simulink model "CPS_PowerSync_System"  (R2024a)
settings: Solver=FixedStepAuto  StartTime=0.0  StopTime=50  FixedStep=0.1  RelTol=1e-3
model workspace (MAT data in the model file):
  SoC : Simulink.Signal (value not decoded)
undefined symbols (not defined in the file or in its folder): m, v_CP1, v_CP2, v_CP3, w_CP1, w_CP2, w_CP3
(part 2 of 3)

== system CPS_PowerSync_System/ElecritcVehicles3/Normal.Plugged.Completed ==
  Action Port : ActionPort
      settings: CopyFcn=Stateflow.SLINSF.SimulinkMan.removeBlockPreDeleteFcn  PreDeleteFcn=Stateflow.SLINSF.SimulinkMan.unsafePredeleteFcn
  Constant : Constant
  If Action Subsystem : Subsystem  TreatAsAtomicUnit=on
  Switch Case : SwitchCase
  plug : Outport
  powerRequest : Outport  Port=2
  wires:
  Constant/1 -> Switch Case/1
  Switch Case/1 -> If Action Subsystem/Action
  If Action Subsystem/1(plug) -> plug/1
  If Action Subsystem/2(powerRequest) -> powerRequest/1

== system CPS_PowerSync_System/ElecritcVehicles3/Normal.Unplugged.Assigment ==
  powerFlow : Inport
  Action Port : ActionPort
      settings: CopyFcn=Stateflow.SLINSF.SimulinkMan.removeBlockPreDeleteFcn  PreDeleteFcn=Stateflow.SLINSF.SimulinkMan.unsafePredeleteFcn
  Constant : Constant  Value=0  OutDataTypeStr=boolean
  powerRequest : Outport
  plug : Outport  Port=2
  wires:
  Constant/1 -> powerRequest/1, plug/1

== system CPS_PowerSync_System/Simulink Function ==
  get_event_CP1 : TriggerPort  TriggerType=function-call  IsSimulinkFunction=on  FunctionName=get_event_CP1  FunctionVisibility=scoped  VariantControl=(inherit)
  Constant : Constant
  Send : Send  OutputPortMessageModes=m
  Out1 : Outport
  wires:
  Constant/1 -> Send/1
  Send/1 -> Out1/1

== system CPS_PowerSync_System/Simulink Function1 ==
  get_event_CP2 : TriggerPort  TriggerType=function-call  IsSimulinkFunction=on  FunctionName=get_event_CP2  FunctionVisibility=scoped  VariantControl=(inherit)
  Constant : Constant
  Send : Send  OutputPortMessageModes=m
  Out1 : Outport
  wires:
  Send/1 -> Out1/1
  Constant/1 -> Send/1

== system CPS_PowerSync_System/Simulink Function2 ==
  dead_CP2 : TriggerPort  TriggerType=function-call  IsSimulinkFunction=on  FunctionName=dead_CP2  FunctionVisibility=scoped  VariantControl=(inherit)
  Constant : Constant  Value=2
  Send : Send  OutputPortMessageModes=m
  Out1 : Outport
  wires:
  Constant/1 -> Send/1
  Send/1 -> Out1/1

== system CPS_PowerSync_System/Simulink Function3 ==
  response_2_to_1 : TriggerPort  TriggerType=function-call  IsSimulinkFunction=on  FunctionName=response_2_to_1  FunctionVisibility=scoped  VariantControl=(inherit)
  Constant : Constant  Value=3
  Send : Send  OutputPortMessageModes=m
  Out1 : Outport
  wires:
  Constant/1 -> Send/1
  Send/1 -> Out1/1

== system CPS_PowerSync_System/Simulink Function4 ==
  response_3_to_2 : TriggerPort  TriggerType=function-call  IsSimulinkFunction=on  FunctionName=response_3_to_2  FunctionVisibility=scoped  VariantControl=(inherit)
  Constant : Constant  Value=3
  Send : Send  OutputPortMessageModes=m
  Out1 : Outport
  wires:
  Send/1 -> Out1/1
  Constant/1 -> Send/1

== system CPS_PowerSync_System/Simulink Function5 ==
  elected_CP3 : TriggerPort  TriggerType=function-call  IsSimulinkFunction=on  FunctionName=elected_CP3  FunctionVisibility=scoped  VariantControl=(inherit)
  Constant : Constant  Value=3
  Send : Send  OutputPortMessageModes=m
  Out1 : Outport
  wires:
  Constant/1 -> Send/1
  Send/1 -> Out1/1

== system CPS_PowerSync_System/Simulink Function6 ==
  elected_CP2 : TriggerPort  TriggerType=function-call  IsSimulinkFunction=on  FunctionName=elected_CP2  FunctionVisibility=scoped  VariantControl=(inherit)
  Constant : Constant  Value=2
  Send : Send  OutputPortMessageModes=m
  Out1 : Outport
  wires:
  Constant/1 -> Send/1
  Send/1 -> Out1/1

== system CPS_PowerSync_System/Simulink Function7 ==
  dead_CP1 : TriggerPort  TriggerType=function-call  IsSimulinkFunction=on  FunctionName=dead_CP1  FunctionVisibility=scoped  VariantControl=(inherit)
  Constant : Constant  Value=2
  Send : Send  OutputPortMessageModes=m
  Out1 : Outport
  wires:
  Constant/1 -> Send/1
  Send/1 -> Out1/1

== system CPS_PowerSync_System/Simulink Function8 ==
  dead_CP3 : TriggerPort  TriggerType=function-call  IsSimulinkFunction=on  FunctionName=dead_CP3  FunctionVisibility=scoped  VariantControl=(inherit)
  Constant : Constant  Value=2
  Send : Send  OutputPortMessageModes=m
  Out1 : Outport
  wires:
  Constant/1 -> Send/1
  Send/1 -> Out1/1

== system CPS_PowerSync_System/Simulink Function9 ==
  response_3_to_1 : TriggerPort  TriggerType=function-call  IsSimulinkFunction=on  FunctionName=response_3_to_1  FunctionVisibility=scoped  VariantControl=(inherit)
  Constant : Constant  Value=3
  Send : Send  OutputPortMessageModes=m
  Out1 : Outport
  wires:
  Constant/1 -> Send/1
  Send/1 -> Out1/1

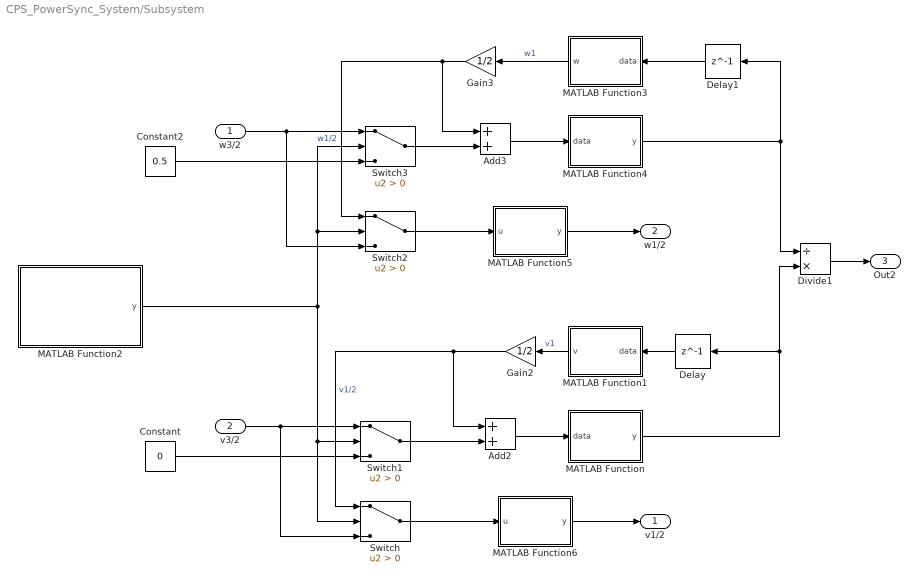
== system CPS_PowerSync_System/Subsystem ==
  w3/2 : Inport  SampleTime=0.1
  v3/2 : Inport  Port=2  SampleTime=0.1
  Add2 : Sum
  Add3 : Sum
  Constant : Constant  Value=0  SampleTime=0.1
  Constant2 : Constant  Value=0.5  SampleTime=0.1
  Delay : Delay  DelayLength=1  InitialCondition=v_CP1  SampleTime=0.1
  Delay1 : Delay  DelayLength=1  InitialCondition=w_CP1  SampleTime=0.1
  Divide1 : Product  Inputs=/*
  Gain2 : Gain  Gain=1/2
  Gain3 : Gain  Gain=1/2
  MATLAB Function : MATLAB Function  TreatAsAtomicUnit=on
  MATLAB Function1 : MATLAB Function  TreatAsAtomicUnit=on
  MATLAB Function2 : MATLAB Function  TreatAsAtomicUnit=on
  MATLAB Function3 : MATLAB Function  TreatAsAtomicUnit=on
  MATLAB Function4 : MATLAB Function  TreatAsAtomicUnit=on
  MATLAB Function5 : MATLAB Function  TreatAsAtomicUnit=on
  MATLAB Function6 : MATLAB Function  TreatAsAtomicUnit=on
  Switch{,1..3} (4 alike) : Switch  Criteria=u2 > Threshold  SaturateOnIntegerOverflow=off  InputSameDT=off
  v1/2 : Outport  SampleTime=0.1
  w1/2 : Outport  Port=2  SampleTime=0.1  VectorParamsAs1DForOutWhenUnconnected=off
  Out2 : Outport  Port=3  OutDataTypeStr=double  SampleTime=0.1
  wires:
  Gain3/1 -> Add3/1, Switch2/1  "w1/2"
  MATLAB Function1/1(v) -> Gain2/1  "v1"
  MATLAB Function2/1(y) -> Switch3/2, Switch2/2, Switch/2, Switch1/2
  Constant/1 -> Switch1/3
  Add3/1 -> MATLAB Function4/1(data)
  v3/2/1 -> Switch1/1, Switch/3
  Switch3/1 -> Add3/2
  MATLAB Function3/1(w) -> Gain3/1  "w1"
  Gain2/1 -> Switch/1, Add2/1  "v1/2"
  Switch1/1 -> Add2/2
  w3/2/1 -> Switch3/1, Switch2/3
  Delay/1 -> MATLAB Function1/1(data)
  Add2/1 -> MATLAB Function/1(data)
  MATLAB Function/1(y) -> Delay/1, Divide1/2
  Divide1/1 -> Out2/1
  Delay1/1 -> MATLAB Function3/1(data)
  MATLAB Function4/1(y) -> Delay1/1, Divide1/1
  Constant2/1 -> Switch3/3
  MATLAB Function5/1(y) -> w1/2/1
  MATLAB Function6/1(y) -> v1/2/1
  Switch2/1 -> MATLAB Function5/1(u)
  Switch/1 -> MATLAB Function6/1(u)

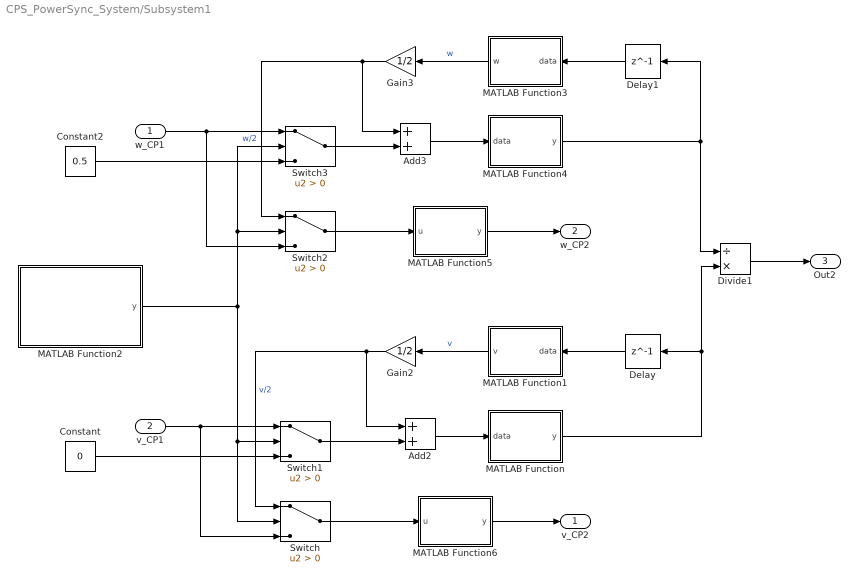
== system CPS_PowerSync_System/Subsystem1 ==
  w_CP1 : Inport  SampleTime=0.1
  v_CP1 : Inport  Port=2  SampleTime=0.1
  Add2 : Sum
  Add3 : Sum
  Constant : Constant  Value=0  SampleTime=0.1
  Constant2 : Constant  Value=0.5  SampleTime=0.1
  Delay : Delay  DelayLength=1  InitialCondition=v_CP2  SampleTime=0.1
  Delay1 : Delay  DelayLength=1  InitialCondition=w_CP2  SampleTime=0.1
  Divide1 : Product  Inputs=/*
  Gain2 : Gain  Gain=1/2
  Gain3 : Gain  Gain=1/2
  MATLAB Function : MATLAB Function  TreatAsAtomicUnit=on
  MATLAB Function1 : MATLAB Function  TreatAsAtomicUnit=on
  MATLAB Function2 : MATLAB Function  TreatAsAtomicUnit=on
  MATLAB Function3 : MATLAB Function  TreatAsAtomicUnit=on
  MATLAB Function4 : MATLAB Function  TreatAsAtomicUnit=on
  MATLAB Function5 : MATLAB Function  TreatAsAtomicUnit=on
  MATLAB Function6 : MATLAB Function  TreatAsAtomicUnit=on
  Switch{,1..3} (4 alike) : Switch  Criteria=u2 > Threshold  SaturateOnIntegerOverflow=off  InputSameDT=off
  v_CP2 : Outport  SampleTime=0.1
  w_CP2 : Outport  Port=2  SampleTime=0.1  VectorParamsAs1DForOutWhenUnconnected=off
  Out2 : Outport  Port=3  OutDataTypeStr=double  SampleTime=0.1
  wires:
  Gain3/1 -> Add3/1, Switch2/1  "w/2"
  MATLAB Function1/1(v) -> Gain2/1  "v"
  MATLAB Function2/1(y) -> Switch3/2, Switch2/2, Switch/2, Switch1/2
  Constant/1 -> Switch1/3
  Add3/1 -> MATLAB Function4/1(data)
  v_CP1/1 -> Switch1/1, Switch/3
  Switch3/1 -> Add3/2
  MATLAB Function3/1(w) -> Gain3/1  "w"
  Gain2/1 -> Switch/1, Add2/1  "v/2"
  Switch1/1 -> Add2/2
  w_CP1/1 -> Switch3/1, Switch2/3
  Delay/1 -> MATLAB Function1/1(data)
  Add2/1 -> MATLAB Function/1(data)
  MATLAB Function/1(y) -> Delay/1, Divide1/2
  Divide1/1 -> Out2/1
  Delay1/1 -> MATLAB Function3/1(data)
  MATLAB Function4/1(y) -> Delay1/1, Divide1/1
  Constant2/1 -> Switch3/3
  MATLAB Function5/1(y) -> w_CP2/1
  MATLAB Function6/1(y) -> v_CP2/1
  Switch2/1 -> MATLAB Function5/1(u)
  Switch/1 -> MATLAB Function6/1(u)

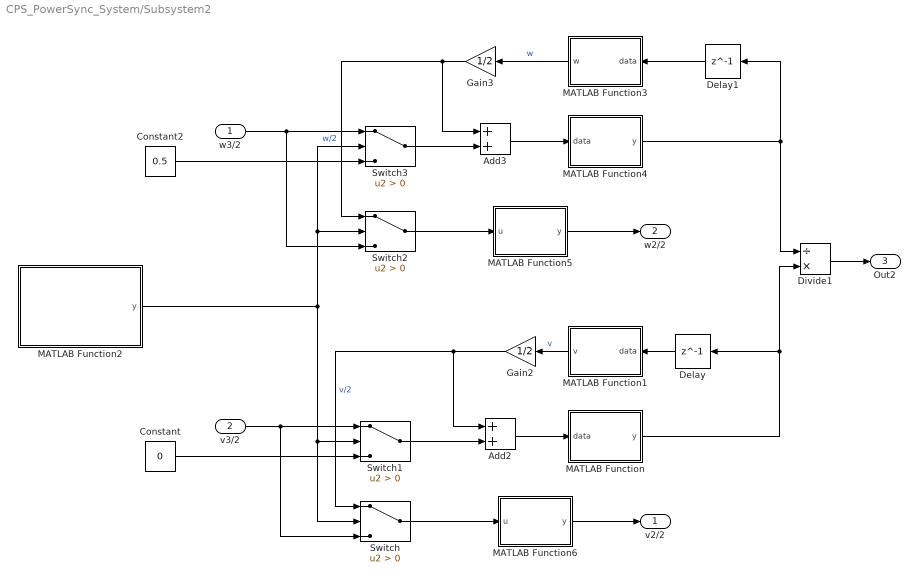
== system CPS_PowerSync_System/Subsystem2 ==
  w3/2 : Inport  SampleTime=0.1
  v3/2 : Inport  Port=2  SampleTime=0.1
  Add2 : Sum
  Add3 : Sum
  Constant : Constant  Value=0  SampleTime=0.1
  Constant2 : Constant  Value=0.5  SampleTime=0.1
  Delay : Delay  DelayLength=1  InitialCondition=v_CP3  SampleTime=0.1
  Delay1 : Delay  DelayLength=1  InitialCondition=w_CP3  SampleTime=0.1
  Divide1 : Product  Inputs=/*
  Gain2 : Gain  Gain=1/2
  Gain3 : Gain  Gain=1/2
  MATLAB Function : MATLAB Function  TreatAsAtomicUnit=on
  MATLAB Function1 : MATLAB Function  TreatAsAtomicUnit=on
  MATLAB Function2 : MATLAB Function  TreatAsAtomicUnit=on
  MATLAB Function3 : MATLAB Function  TreatAsAtomicUnit=on
  MATLAB Function4 : MATLAB Function  TreatAsAtomicUnit=on
  MATLAB Function5 : MATLAB Function  TreatAsAtomicUnit=on
  MATLAB Function6 : MATLAB Function  TreatAsAtomicUnit=on
  Switch{,1..3} (4 alike) : Switch  Criteria=u2 > Threshold  SaturateOnIntegerOverflow=off  InputSameDT=off
  v2/2 : Outport  SampleTime=0.1
  w2/2 : Outport  Port=2  SampleTime=0.1  VectorParamsAs1DForOutWhenUnconnected=off
  Out2 : Outport  Port=3  OutDataTypeStr=double  SampleTime=0.1
  wires:
  Gain3/1 -> Add3/1, Switch2/1  "w/2"
  MATLAB Function1/1(v) -> Gain2/1  "v"
  MATLAB Function2/1(y) -> Switch3/2, Switch2/2, Switch/2, Switch1/2
  Constant/1 -> Switch1/3
  Add3/1 -> MATLAB Function4/1(data)
  v3/2/1 -> Switch1/1, Switch/3
  Switch3/1 -> Add3/2
  MATLAB Function3/1(w) -> Gain3/1  "w"
  Gain2/1 -> Switch/1, Add2/1  "v/2"
  Switch1/1 -> Add2/2
  w3/2/1 -> Switch3/1, Switch2/3
  Delay/1 -> MATLAB Function1/1(data)
  Add2/1 -> MATLAB Function/1(data)
  MATLAB Function/1(y) -> Delay/1, Divide1/2
  Divide1/1 -> Out2/1
  Delay1/1 -> MATLAB Function3/1(data)
  MATLAB Function4/1(y) -> Delay1/1, Divide1/1
  Constant2/1 -> Switch3/3
  MATLAB Function5/1(y) -> w2/2/1
  MATLAB Function6/1(y) -> v2/2/1
  Switch2/1 -> MATLAB Function5/1(u)
  Switch/1 -> MATLAB Function6/1(u)

== system CPS_PowerSync_System/WirelessReceiveModule ==
  Bus Selector : BusSelector  OutputSignals=v3/2,w3/2
  Multicast Receive Queue : Queue  OutputPortMessageModes=m  EntityArrivalSource=Multicast  MulticastTag=F
  Receive : Receive  InputPortMessageModes=m  UseInternalQueue=off  QueueOverwriting=on  QueueLength=1  QueueType=LIFO  SampleTime=0.1
  <w3/2> : Outport  SampleTime=0.1
  <v3/2> : Outport  Port=2  SampleTime=0.1
  wires:
  Receive/1 -> Bus Selector/1
  Bus Selector/1 -> <v3/2>/1  "<v3/2>"
  Bus Selector/2 -> <w3/2>/1  "<w3/2>"
  Multicast Receive Queue/1 -> Receive/1

== system CPS_PowerSync_System/WirelessReceiveModule1 ==
  Bus Selector : BusSelector  OutputSignals=w1/2,v1/2
  Multicast Receive Queue : Queue  OutputPortMessageModes=m  EntityArrivalSource=Multicast  MulticastTag=D
  Receive : Receive  InputPortMessageModes=m  UseInternalQueue=off  QueueOverwriting=on  QueueLength=1  QueueType=LIFO
  <w1/2> : Outport  SampleTime=0.1
  <v1/2> : Outport  Port=2  SampleTime=0.1
  wires:
  Bus Selector/2 -> <v1/2>/1  "<v1/2>"
  Multicast Receive Queue/1 -> Receive/1
  Receive/1 -> Bus Selector/1
  Bus Selector/1 -> <w1/2>/1  "<w1/2>"

== system CPS_PowerSync_System/WirelessReceiveModule2 ==
  Bus Selector : BusSelector  OutputSignals=v2/2,w2/2
  Multicast Receive Queue : Queue  OutputPortMessageModes=m  EntityArrivalSource=Multicast  MulticastTag=E
  Receive : Receive  InputPortMessageModes=m  UseInternalQueue=off  QueueOverwriting=on  QueueLength=1  QueueType=LIFO
  <w2/2> : Outport  SampleTime=0.1
  <v2/2> : Outport  Port=2  SampleTime=0.1
  wires:
  Bus Selector/2 -> <w2/2>/1  "<w2/2>"
  Multicast Receive Queue/1 -> Receive/1
  Receive/1 -> Bus Selector/1
  Bus Selector/1 -> <v2/2>/1  "<v2/2>"

== system CPS_PowerSync_System/WirelessSendModule ==
  v1/2 : Inport  SampleTime=0.1
  w1/2 : Inport  Port=2  SampleTime=0.1
  Bus Creator : BusCreator  Inputs=2  OutDataTypeStr=Bus: BusObject  NonVirtualBus=on
  Entity Multicast : EntityMulticast  Tag=D  InputPortMessageModes=m  MulticastTag=D
  Send : Send  OutputPortMessageModes=m
  wires:
  Send/1 -> Entity Multicast/1
  Bus Creator/1 -> Send/1
  v1/2/1 -> Bus Creator/2  "v1/2"
  w1/2/1 -> Bus Creator/1  "w1/2"

== system CPS_PowerSync_System/WirelessSendModule1 ==
  v2/2 : Inport  SampleTime=0.1
  w2/2 : Inport  Port=2  SampleTime=0.1
  Bus Creator : BusCreator  Inputs=2  OutDataTypeStr=Bus: BusObject  NonVirtualBus=on
  Entity Multicast : EntityMulticast  Tag=E  InputPortMessageModes=m  MulticastTag=E
  Send : Send  OutputPortMessageModes=m
  wires:
  Bus Creator/1 -> Send/1
  Send/1 -> Entity Multicast/1
  v2/2/1 -> Bus Creator/1  "v2/2"
  w2/2/1 -> Bus Creator/2  "w2/2"

== system CPS_PowerSync_System/WirelessSendModule2 ==
  v3/2 : Inport  SampleTime=0.1
  w3/2 : Inport  Port=2  SampleTime=0.1
  Bus Creator : BusCreator  Inputs=2  OutDataTypeStr=Bus: BusObject  NonVirtualBus=on
  Entity Multicast : EntityMulticast  Tag=F  InputPortMessageModes=m  MulticastTag=F
  Send : Send  OutputPortMessageModes=m
  wires:
  Bus Creator/1 -> Send/1
  v3/2/1 -> Bus Creator/1  "v3/2"
  w3/2/1 -> Bus Creator/2  "w3/2"
  Send/1 -> Entity Multicast/1

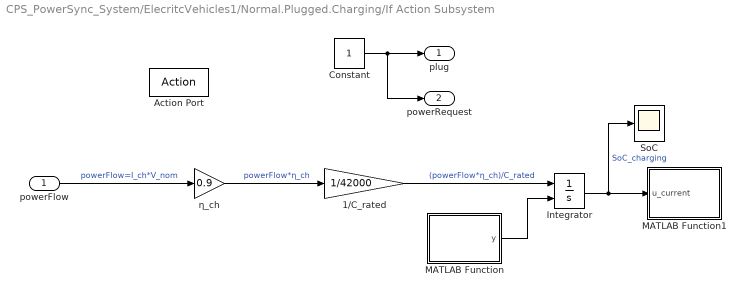
== system CPS_PowerSync_System/ElecritcVehicles1/Normal.Plugged.Charging/If Action Subsystem ==
  powerFlow : Inport
  Action Port : ActionPort  InitializeStates=reset  ActionPortLabel=case [ 1 ]:
  1/C_rated : Gain  Gain=1/42000
  Constant : Constant  OutDataTypeStr=boolean
  Integrator : Integrator  InitialConditionSource=external  LimitOutput=on  UpperSaturationLimit=1  LowerSaturationLimit=0
  MATLAB Function : MATLAB Function  TreatAsAtomicUnit=on
  MATLAB Function1 : MATLAB Function  TreatAsAtomicUnit=on
  SoC : Scope
  η_ch : Gain  Gain=0.9
  plug : Outport  OutDataTypeStr=boolean
  powerRequest : Outport  Port=2  OutDataTypeStr=boolean
  wires:
  1/C_rated/1 -> Integrator/1  "(powerFlow*η_ch)/C_rated"
  η_ch/1 -> 1/C_rated/1  "powerFlow*η_ch"
  Constant/1 -> plug/1, powerRequest/1
  Integrator/1 -> SoC/1, MATLAB Function1/1(u_current)  "SoC_charging"
  powerFlow/1 -> η_ch/1  "powerFlow=I_ch*V_nom"
  MATLAB Function/1(y) -> Integrator/2

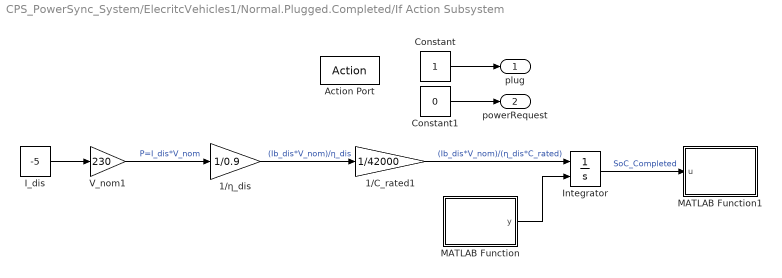
== system CPS_PowerSync_System/ElecritcVehicles1/Normal.Plugged.Completed/If Action Subsystem ==
  Action Port : ActionPort  InitializeStates=reset  ActionPortLabel=case [ 1 ]:
  1/C_rated1 : Gain  Gain=1/42000
  1/η_dis : Gain  Gain=1/0.9
  Constant : Constant  OutDataTypeStr=boolean
  Constant1 : Constant  Value=0  OutDataTypeStr=boolean
  I_dis : Constant  Value=-5
  Integrator : Integrator  InitialConditionSource=external  LimitOutput=on  UpperSaturationLimit=1  LowerSaturationLimit=0
  MATLAB Function : MATLAB Function  TreatAsAtomicUnit=on
  MATLAB Function1 : MATLAB Function  TreatAsAtomicUnit=on
  V_nom1 : Gain  Gain=230
  plug : Outport  OutDataTypeStr=boolean
  powerRequest : Outport  Port=2  OutDataTypeStr=boolean
  wires:
  Integrator/1 -> MATLAB Function1/1(u)  "SoC_Completed"
  MATLAB Function/1(y) -> Integrator/2
  Constant1/1 -> powerRequest/1
  1/η_dis/1 -> 1/C_rated1/1  "(Ib_dis*V_nom)/η_dis"
  V_nom1/1 -> 1/η_dis/1  "P=I_dis*V_nom"
  1/C_rated1/1 -> Integrator/1  "(Ib_dis*V_nom)/(η_dis*C_rated)"
  I_dis/1 -> V_nom1/1
  Constant/1 -> plug/1

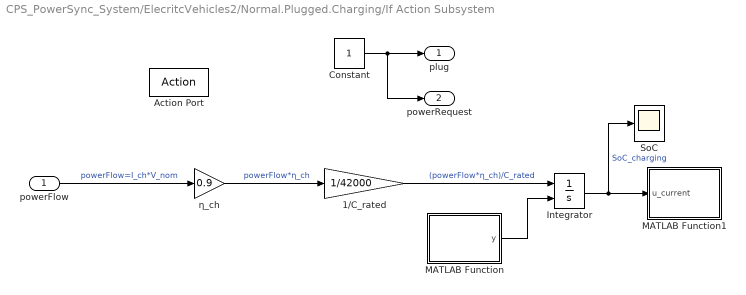
== system CPS_PowerSync_System/ElecritcVehicles2/Normal.Plugged.Charging/If Action Subsystem ==
  powerFlow : Inport
  Action Port : ActionPort  InitializeStates=reset  ActionPortLabel=case [ 1 ]:
  1/C_rated : Gain  Gain=1/42000
  Constant : Constant  OutDataTypeStr=boolean
  Integrator : Integrator  InitialConditionSource=external  LimitOutput=on  UpperSaturationLimit=1  LowerSaturationLimit=0
  MATLAB Function : MATLAB Function  TreatAsAtomicUnit=on
  MATLAB Function1 : MATLAB Function  TreatAsAtomicUnit=on
  SoC : Scope
  η_ch : Gain  Gain=0.9
  plug : Outport  OutDataTypeStr=boolean
  powerRequest : Outport  Port=2  OutDataTypeStr=boolean
  wires:
  MATLAB Function/1(y) -> Integrator/2
  powerFlow/1 -> η_ch/1  "powerFlow=I_ch*V_nom"
  Integrator/1 -> MATLAB Function1/1(u_current), SoC/1  "SoC_charging"
  Constant/1 -> powerRequest/1, plug/1
  η_ch/1 -> 1/C_rated/1  "powerFlow*η_ch"
  1/C_rated/1 -> Integrator/1  "(powerFlow*η_ch)/C_rated"

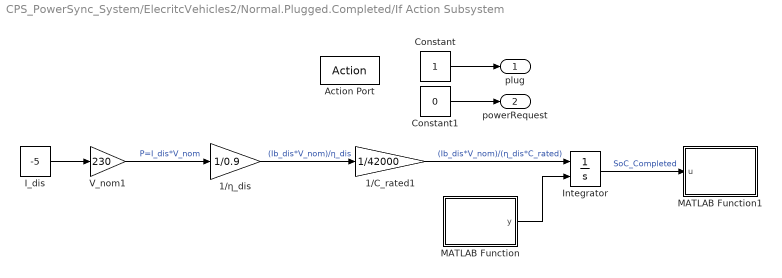
== system CPS_PowerSync_System/ElecritcVehicles2/Normal.Plugged.Completed/If Action Subsystem ==
  Action Port : ActionPort  InitializeStates=reset  ActionPortLabel=case [ 1 ]:
  1/C_rated1 : Gain  Gain=1/42000
  1/η_dis : Gain  Gain=1/0.9
  Constant : Constant  OutDataTypeStr=boolean
  Constant1 : Constant  Value=0  OutDataTypeStr=boolean
  I_dis : Constant  Value=-5
  Integrator : Integrator  InitialConditionSource=external  LimitOutput=on  UpperSaturationLimit=1  LowerSaturationLimit=0
  MATLAB Function : MATLAB Function  TreatAsAtomicUnit=on
  MATLAB Function1 : MATLAB Function  TreatAsAtomicUnit=on
  V_nom1 : Gain  Gain=230
  plug : Outport  OutDataTypeStr=boolean
  powerRequest : Outport  Port=2  OutDataTypeStr=boolean
  wires:
  Constant/1 -> plug/1
  I_dis/1 -> V_nom1/1
  1/C_rated1/1 -> Integrator/1  "(Ib_dis*V_nom)/(η_dis*C_rated)"
  V_nom1/1 -> 1/η_dis/1  "P=I_dis*V_nom"
  1/η_dis/1 -> 1/C_rated1/1  "(Ib_dis*V_nom)/η_dis"
  Constant1/1 -> powerRequest/1
  MATLAB Function/1(y) -> Integrator/2
  Integrator/1 -> MATLAB Function1/1(u)  "SoC_Completed"

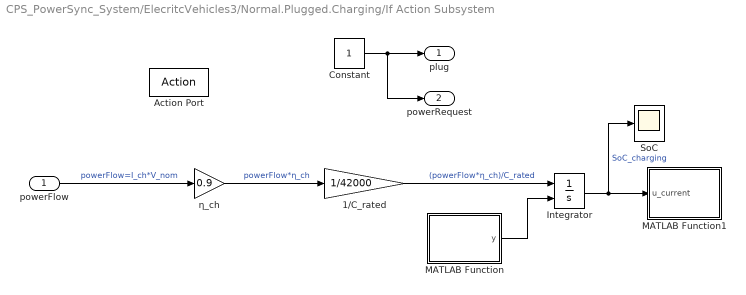
== system CPS_PowerSync_System/ElecritcVehicles3/Normal.Plugged.Charging/If Action Subsystem ==
  powerFlow : Inport
  Action Port : ActionPort  InitializeStates=reset  ActionPortLabel=case [ 1 ]:
  1/C_rated : Gain  Gain=1/42000
  Constant : Constant  OutDataTypeStr=boolean
  Integrator : Integrator  InitialConditionSource=external  LimitOutput=on  UpperSaturationLimit=1  LowerSaturationLimit=0
  MATLAB Function : MATLAB Function  TreatAsAtomicUnit=on
  MATLAB Function1 : MATLAB Function  TreatAsAtomicUnit=on
  SoC : Scope
  η_ch : Gain  Gain=0.9
  plug : Outport  OutDataTypeStr=boolean
  powerRequest : Outport  Port=2  OutDataTypeStr=boolean
  wires:
  1/C_rated/1 -> Integrator/1  "(powerFlow*η_ch)/C_rated"
  η_ch/1 -> 1/C_rated/1  "powerFlow*η_ch"
  Constant/1 -> plug/1, powerRequest/1
  Integrator/1 -> SoC/1, MATLAB Function1/1(u_current)  "SoC_charging"
  powerFlow/1 -> η_ch/1  "powerFlow=I_ch*V_nom"
  MATLAB Function/1(y) -> Integrator/2

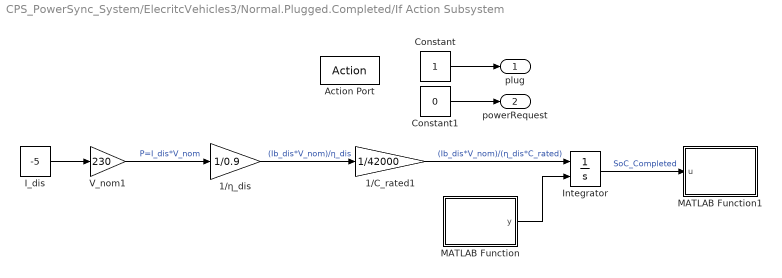
== system CPS_PowerSync_System/ElecritcVehicles3/Normal.Plugged.Completed/If Action Subsystem ==
  Action Port : ActionPort  InitializeStates=reset  ActionPortLabel=case [ 1 ]:
  1/C_rated1 : Gain  Gain=1/42000
  1/η_dis : Gain  Gain=1/0.9
  Constant : Constant  OutDataTypeStr=boolean
  Constant1 : Constant  Value=0  OutDataTypeStr=boolean
  I_dis : Constant  Value=-5
  Integrator : Integrator  InitialConditionSource=external  LimitOutput=on  UpperSaturationLimit=1  LowerSaturationLimit=0
  MATLAB Function : MATLAB Function  TreatAsAtomicUnit=on
  MATLAB Function1 : MATLAB Function  TreatAsAtomicUnit=on
  V_nom1 : Gain  Gain=230
  plug : Outport  OutDataTypeStr=boolean
  powerRequest : Outport  Port=2  OutDataTypeStr=boolean
  wires:
  Integrator/1 -> MATLAB Function1/1(u)  "SoC_Completed"
  MATLAB Function/1(y) -> Integrator/2
  Constant1/1 -> powerRequest/1
  1/η_dis/1 -> 1/C_rated1/1  "(Ib_dis*V_nom)/η_dis"
  V_nom1/1 -> 1/η_dis/1  "P=I_dis*V_nom"
  1/C_rated1/1 -> Integrator/1  "(Ib_dis*V_nom)/(η_dis*C_rated)"
  I_dis/1 -> V_nom1/1
  Constant/1 -> plug/1

== matlab function CPS_PowerSync_System/CP1 ==
  settings: updateMethod=DISCRETE  sampleTime=0.1
  data: clock input
function fcn(clock)

    % Funzioni per interagire con base workspace
    coder.extrinsic('evalin');
    coder.extrinsic('assignin');
    
    check_variables('flg_response_CP1');
    check_variables('t_send_CP1');
    check_variables('flg_send_CP1');
    check_variables('pr_previous_CP1');
    check_variables('pr_actual_CP1');
    
    % Aggiornamento del clock del CP1
    assignin('base', 'clock_CP1', clock);
    
    % Lettura variabili dal WS
    pr_previous = boolean(0); pr_actual = boolean(0); t_send = 0;
    pr_previous = evalin('base', 'boolean(pr_previous_CP1)');
    pr_actual = evalin('base', 'boolean(pr_actual_CP1)');
    t_send = evalin('base', 'double(t_send_CP1)');
    flg_response = evalin('base', 'boolean(flg_response_CP1)');
    flg_send = evalin('base', 'boolean(flg_send_CP1)');


    % Controllo se un veicolo si è connesso / disconnesso
    if pr_previous ~= pr_actual

        if pr_actual
            disp('CP1 requires power, so the leader must be re-elected.')
        else
            disp('CP1 requires no additional power, so the leader must be re-elected.')
        end
        
        dead_CP1();

    end

    % Controllo se mi è possibile diventare leader:

    % Tempo trascorso dall'invio del messaggio da parte del nodo 1
    t_elapsed = clock - t_send; 

    % Definizione del tempo da attendere per elezione leader
    delta = 1;
    
    % Se dopo delta secondi dal momento in cui ho inviato il messaggio
    % (t_elapsed >= delta) non ho ancora ricevuto una risposta
    % (~flg_response) e il mio flag_inviato non è stato resettato a zero
    % e ho il veicolo connesso, allora sarò il leader
    if t_elapsed >= delta && ~flg_response && flg_send && pr_actual

        % Il nodo 1 diventa leader
        assignin('base', 'v_CP1', 1);

        % Il nodo sa che il leader è stato eletto
        assignin('base', 'flg_elected_CP1', 1);

        disp('CP1 did not receive an answer, so it can declare itself leader.')

        % Elezione avvenuta
        % Tutti e tre questi flag sono necessari al corretto funzionamento dell'algoritmo push-sum
        assignin('base', 'flg_elected_CP1', 1);
        assignin('base', 'flg_first_instant_v_CP1', 1);
        assignin('base', 'flg_first_instant_w_CP1', 1);
    
        assignin('base', 'flg_send_CP1', 0);
        
        disp('CP1 is active and knows that the leader has been elected.')
        
    end

end

== matlab function CPS_PowerSync_System/CP2 ==
  settings: updateMethod=DISCRETE  sampleTime=0.1
  data: clock input
function fcn(clock)

    % Funzioni per interagire con base workspace
    coder.extrinsic('evalin');
    coder.extrinsic('assignin');
    
    check_variables('flg_response_CP2');
    check_variables('t_send_CP2');
    check_variables('flg_send_CP2');
    check_variables('pr_previous_CP2');
    check_variables('pr_actual_CP2');
    
    % Aggiornamento del clock del CP2
    assignin('base', 'clock_CP2', clock);
    
    % Lettura variabili dal WS
    pr_previous = boolean(0); pr_actual = boolean(0); t_send = 0;
    pr_previous = evalin('base', 'boolean(pr_previous_CP2)');
    pr_actual = evalin('base', 'boolean(pr_actual_CP2)');
    t_send = evalin('base', 'double(t_send_CP2)');
    flg_response = evalin('base', 'boolean(flg_response_CP2)');
    flg_send = evalin('base', 'boolean(flg_send_CP2)');


    % Controllo se un veicolo si è connesso / disconnesso
    if pr_previous ~= pr_actual

        if pr_actual
            disp('CP2 requires power, so the leader must be re-elected.')
        else
            disp('CP2 requires no additional power, so the leader must be re-elected.')
        end
        
        dead_CP2();

    end

    % Controllo se mi è possibile diventare leader:

    % Tempo trascorso dall'invio del messaggio da parte del nodo 1
    t_elapsed = clock - t_send; 

    % Definizione del tempo da attendere per elezione leader
    delta = 1;
    
    % Se dopo delta secondi dal momento in cui ho inviato il messaggio
    % (t_elapsed >= delta) non ho ancora ricevuto una risposta
    % (~flg_response) e il mio flag_inviato non è stato resettato a zero
    % e ho il veicolo connesso, allora sarò il leader
    if t_elapsed >= delta && ~flg_response && flg_send && pr_actual

        % Il nodo 1 diventa leader
        assignin('base', 'v_CP2', 1);

        % Il nodo sa che il leader è stato eletto
        assignin('base', 'flg_elected_CP2', 1);

        disp('CP2 did not receive an answer, so it can declare itself leader.')

        % Notifico agli altri l'elezione
        elected_CP2();
        
    end

end

== stateflow chart CPS_PowerSync_System/ElecritcVehicles1 ==
  settings: updateMethod=CONTINUOUS  sampleTime=1
  state Normal
    entry:
    % Imposto generatore casuali in dtato basato su ora corrente
    rng("shuffle")
    % Imposto casualmente valore iniziale di SoC
    SoC_EV1 = randi([0,10])/10
    state Unplugged
      state Assigment
    state Plugged
      state Charging
      state Completed
      (default) -> (junction 33)
      (junction 33) -> Charging [order 2]
      (junction 33) -> Completed [order 1] : [SoC_EV1 == 1]
      Completed -> Charging : [SoC_EV1 <= 0.95]
      Charging -> Completed : [SoC_EV1 == 1]
    (default) -> Unplugged
    Unplugged -> Plugged : [runPythonScriptRandGen <= (1 - exp((-(elapsed(sec))/10)))]
    Plugged -> Unplugged : % Il veicolo si scollega e se ne collega un altro
        | % P1: Maggiore è il valore di SoC più è probabile che il veicolo se ne vada
        | % P2: La proabilità che il veicolo se ne vada aumenta con il passare del tempo
        | [runPythonScriptRandGen <= SoC_EV1 && runPythonScriptRandGen <= (1 - exp((-(elapsed(sec))/100)))]
        | {% Arriva nuovo veicolo con un proprio valore di SoC
        |  SoC_EV1 = randi([0,10])/10}
  (default) -> Normal
  data: sf_internal_action_state_placeholder_data local double size=1 =0; randUniform function_output; sf_internal_action_state_placeholder_data local double size=1 =0; sf_internal_action_state_placeholder_data local double size=1 =0; powerFlow input double; powerRequest output boolean =0; plug output boolean size=1; SoC_EV1 data_store_memory
  function randUniform = runPythonScriptRandGen:
    | function randUniform = runPythonScriptRandGen()
    | 
    |     % La funzione è estrinseca, cioè non verrà compilata in codice C.
    |     % Deve essere eseguita come una chiamata MATLAB normale.
    |     coder.extrinsic('pyrunfile');
    | 
    |     % Inizializzo la variabile
    |     randUniform = 0;
    | 
    |     % Esegue lo script Python rand.py e cattura il risultato.
    |     randUniform = pyrunfile("rand.py", "r");
    | 
    | end

== matlab function CPS_PowerSync_System/CP3 ==
  settings: updateMethod=DISCRETE  sampleTime=0.1
  data: clock input
function fcn(clock)

    % Funzioni per interagire con base workspace
    coder.extrinsic('evalin');
    coder.extrinsic('assignin');
    
    check_variables('flg_response_CP3');
    check_variables('t_send_CP3');
    check_variables('flg_send_CP3');
    check_variables('pr_previous_CP3');
    check_variables('pr_actual_CP3');
    
    % Aggiornamento del clock del CP3
    assignin('base', 'clock_CP3', clock);
    
    % Lettura variabili dal WS
    pr_previous = boolean(0); pr_actual = boolean(0); t_send = 0;
    pr_previous = evalin('base', 'boolean(pr_previous_CP3)');
    pr_actual = evalin('base', 'boolean(pr_actual_CP3)');
    t_send = evalin('base', 'double(t_send_CP3)');
    flg_response = evalin('base', 'boolean(flg_response_CP3)');
    flg_send = evalin('base', 'boolean(flg_send_CP3)');


    % Controllo se un veicolo si è connesso / disconnesso
    if pr_previous ~= pr_actual

        if pr_actual
            disp('CP3 requires power, so the leader must be re-elected.')
        else
            disp('CP3 requires no additional power, so the leader must be re-elected.')
        end
        
        dead_CP3();

    end

    % Controllo se mi è possibile diventare leader:

    % Tempo trascorso dall'invio del messaggio da parte del nodo 1
    t_elapsed = clock - t_send; 

    % Definizione del tempo da attendere per elezione leader
    delta = 1;
    
    % Se dopo delta secondi dal momento in cui ho inviato il messaggio
    % (t_elapsed >= delta) non ho ancora ricevuto una risposta
    % (~flg_response) e il mio flag_inviato non è stato resettato a zero
    % e ho il veicolo connesso, allora sarò il leader
    if t_elapsed >= delta && ~flg_response && flg_send && pr_actual

        % Il nodo 1 diventa leader
        assignin('base', 'v_CP3', 1);

        % Il nodo sa che il leader è stato eletto
        assignin('base', 'flg_elected_CP3', 1);

        disp('CP3 did not receive an answer, so it can declare itself leader.')

        % Notifico agli altri l'elezione
        elected_CP3();
        
    end

end

== stateflow chart CPS_PowerSync_System/ChargingPoint2 ==
  settings: updateMethod=CONTINUOUS  sampleTime=1
  state Normal
    state Idle
      state Assignment
    state Connected
      state Powering
        state Assignment
      state NotPowering
        state Assignment
      (default) -> (junction 23)
      (junction 23) -> Powering [order 1] : [powerRequest == 1]
      (junction 23) -> NotPowering [order 2]
      NotPowering -> Powering : [powerRequest == 1]
      Powering -> NotPowering : [powerRequest == 0]
    (default) -> (junction 31)
    (junction 31) -> Idle [order 1] : [plug == 0]
    (junction 31) -> Connected [order 2]
    Connected -> Idle : [plug == 0]
    Idle -> Connected : [plug == 1]
  state Error
    state Assignment
  (default) -> Normal
  Normal -> Error : [runPythonScriptRandGen <= (1 - exp((-(elapsed(sec))/300)))]
  Error -> Normal : after(10,sec)
  data: sf_internal_action_state_placeholder_data local double size=1 =0; sf_internal_action_state_placeholder_data local double size=1 =0; sf_internal_action_state_placeholder_data local double size=1 =0; sf_internal_action_state_placeholder_data local double size=1 =0; randUniform function_output; enablePowerFlow output boolean; powerRequest input boolean; plug input boolean
  function randUniform = runPythonScriptRandGen:
    | function randUniform = runPythonScriptRandGen()
    | 
    |     % La funzione è estrinseca, cioè non verrà compilata in codice C.
    |     % Deve essere eseguita come una chiamata MATLAB normale.
    |     coder.extrinsic('pyrunfile');
    | 
    |     % Inizializzo la variabile
    |     randUniform = 0;
    | 
    |     % Esegue lo script Python rand.py e cattura il risultato.
    |     randUniform = pyrunfile("rand.py", "r");
    | end

== stateflow chart CPS_PowerSync_System/ChargingPoint3 ==
  settings: updateMethod=CONTINUOUS  sampleTime=1
  state Normal
    state Idle
      state Assignment
    state Connected
      state Powering
        state Assignment
      state NotPowering
        state Assignment
      (default) -> (junction 23)
      (junction 23) -> Powering [order 1] : [powerRequest == 1]
      (junction 23) -> NotPowering [order 2]
      NotPowering -> Powering : [powerRequest == 1]
      Powering -> NotPowering : [powerRequest == 0]
    (default) -> (junction 31)
    (junction 31) -> Idle [order 1] : [plug == 0]
    (junction 31) -> Connected [order 2]
    Connected -> Idle : [plug == 0]
    Idle -> Connected : [plug == 1]
  state Error
    state Assignment
  (default) -> Normal
  Normal -> Error : [runPythonScriptRandGen <= (1 - exp((-(elapsed(sec))/300)))]
  Error -> Normal : after(10,sec)
  data: sf_internal_action_state_placeholder_data local double size=1 =0; sf_internal_action_state_placeholder_data local double size=1 =0; sf_internal_action_state_placeholder_data local double size=1 =0; sf_internal_action_state_placeholder_data local double size=1 =0; randUniform function_output; enablePowerFlow output boolean; powerRequest input boolean; plug input boolean
  function randUniform = runPythonScriptRandGen:
    | function randUniform = runPythonScriptRandGen()
    | 
    |     % La funzione è estrinseca, cioè non verrà compilata in codice C.
    |     % Deve essere eseguita come una chiamata MATLAB normale.
    |     coder.extrinsic('pyrunfile');
    | 
    |     % Inizializzo la variabile
    |     randUniform = 0;
    | 
    |     % Esegue lo script Python rand.py e cattura il risultato.
    |     randUniform = pyrunfile("rand.py", "r");
    | end

== matlab function CPS_PowerSync_System/Subsystem/MATLAB Function1 ==
  settings: updateMethod=DISCRETE  sampleTime=0.1
  data: v output; data input
function v = readVariable(data)

    coder.extrinsic('evalin');

    v = 0;

    flag_elected = 0;
    flag_elected = evalin('base', 'flg_elected_CP1'); % Legge la variabile v1 dal Base Workspace

    flag_first_instant = 0;
    flag_first_instant = evalin('base', 'flg_first_instant_v_CP1'); % Legge la variabile v1 dal Base Workspace


    % CI DEVI ANDARE SOLO LA PRIMA VOLTA 
    if flag_elected == 1 && flag_first_instant == 1
        v = evalin('base', 'v_CP1');
        assignin('base', 'flg_first_instant_v_CP1', 0);
    else
        assignin('base', 'v_CP1', data);
        v = data;
    end

end

== matlab function CPS_PowerSync_System/Subsystem/MATLAB Function2 ==
  settings: updateMethod=DISCRETE  sampleTime=0.1
  data: y output
function y = fcn()

    y = 0;
    coder.extrinsic('evalin');

    flag_elected = 0;
    flag_elected = evalin('base', 'flg_elected_CP1');

    if flag_elected == 0
        % Significa che il CP 2 non partecipa e deve solo fare da
        % intermediario
        y = 0;
    else if flag_elected == 1
            % Il leader esiste (potrebbe essere il 2 o il 3)
            y = 1;
        end
    end
   
end

== stateflow chart CPS_PowerSync_System/ElecritcVehicles2 ==
  settings: updateMethod=CONTINUOUS  sampleTime=1
  state Normal
    entry:
    % Imposto generatore casuali in dtato basato su ora corrente
    rng("shuffle")
    % Imposto casualmente valore iniziale di SoC
    SoC_EV2 = randi([0,10])/10
    state Unplugged
      state Assigment
    state Plugged
      state Charging
      state Completed
      (default) -> (junction 33)
      (junction 33) -> Charging [order 2]
      (junction 33) -> Completed [order 1] : [SoC_EV2 == 1]
      Completed -> Charging : [SoC_EV2 <= 0.95]
      Charging -> Completed : [SoC_EV2 == 1]
    (default) -> Unplugged
    Unplugged -> Plugged : [runPythonScriptRandGen <= (1 - exp((-(elapsed(sec))/10)))]
    Plugged -> Unplugged : % Il veicolo si scollega e se ne collega un altro
        | % P1: Maggiore è il valore di SoC più è probabile che il veicolo se ne vada
        | % P2: La proabilità che il veicolo se ne vada aumenta con il passare del tempo
        | [runPythonScriptRandGen <= SoC_EV2 && runPythonScriptRandGen <= (1 - exp((-(elapsed(sec))/100)))]
        | {% Arriva nuovo veicolo con un proprio valore di SoC
        |  SoC_EV2 = randi([0,10])/10}
  (default) -> Normal
  data: sf_internal_action_state_placeholder_data local double size=1 =0; randUniform function_output; sf_internal_action_state_placeholder_data local double size=1 =0; sf_internal_action_state_placeholder_data local double size=1 =0; powerFlow input double; powerRequest output boolean =0; plug output boolean size=1; SoC_EV2 data_store_memory
  function randUniform = runPythonScriptRandGen:
    | function randUniform = runPythonScriptRandGen()
    | 
    |     % La funzione è estrinseca, cioè non verrà compilata in codice C.
    |     % Deve essere eseguita come una chiamata MATLAB normale.
    |     coder.extrinsic('pyrunfile');
    | 
    |     % Inizializzo la variabile
    |     randUniform = 0;
    | 
    |     % Esegue lo script Python rand.py e cattura il risultato.
    |     randUniform = pyrunfile("rand.py", "r");
    | 
    | end

== matlab function CPS_PowerSync_System/Subsystem2/MATLAB Function ==
  settings: updateMethod=DISCRETE  sampleTime=0.1
  data: y output; data input
function y = fcn(data)

    coder.extrinsic('evalin');

    flag_dead = 0;
    flag_dead = evalin('base', 'flg_dead_v_CP3');

    if flag_dead == 1
        y = 0;
        assignin('base', 'flg_dead_v_CP3', 0);
    else
        y = data;
    end

end

== matlab function CPS_PowerSync_System/Subsystem1/MATLAB Function ==
  settings: updateMethod=DISCRETE  sampleTime=0.1
  data: y output; data input
function y = fcn(data)

    coder.extrinsic('evalin');

    flag_dead = 0;
    flag_dead = evalin('base', 'flg_dead_v_CP2');

    if flag_dead == 1
        y = 0;
        assignin('base', 'flg_dead_v_CP2', 0);
    else
        y = data;
    end

end

== matlab function CPS_PowerSync_System/Subsystem1/MATLAB Function1 ==
  settings: updateMethod=DISCRETE  sampleTime=0.1
  data: v output; data input
function v = readVariable(data)

    coder.extrinsic('evalin');

    v = 0;

    flag_elected = 0;
    flag_elected = evalin('base', 'flg_elected_CP2'); % Legge la variabile v1 dal Base Workspace

    flag_first_instant = 0;
    flag_first_instant = evalin('base', 'flg_first_instant_v_CP2'); % Legge la variabile v1 dal Base Workspace


    % CI DEVI ANDARE SOLO LA PRIMA VOLTA 
    if flag_elected == 1 && flag_first_instant == 1
        v = evalin('base', 'v_CP2');
        assignin('base', 'flg_first_instant_v_CP2', 0);
    else
        assignin('base', 'v_CP2', data);
        v = data;
    end

end

== matlab function CPS_PowerSync_System/Subsystem2/MATLAB Function1 ==
  settings: updateMethod=DISCRETE  sampleTime=0.1
  data: v output; data input
function v = readVariable(data)

    coder.extrinsic('evalin');

    v = 0;

    flag_elected = 0;
    flag_elected = evalin('base', 'flg_elected_CP3'); % Legge la variabile v1 dal Base Workspace

    flag_first_instant = 0;
    flag_first_instant = evalin('base', 'flg_first_instant_v_CP3'); % Legge la variabile v1 dal Base Workspace


    % CI DEVI ANDARE SOLO LA PRIMA VOLTA 
    if flag_elected == 1 && flag_first_instant == 1
        v = evalin('base', 'v_CP3');
        assignin('base', 'flg_first_instant_v_CP3', 0);
    else
        assignin('base', 'v_CP3', data);
        v = data;
    end

end

== matlab function CPS_PowerSync_System/Subsystem/MATLAB Function ==
  settings: updateMethod=DISCRETE  sampleTime=0.1
  data: y output; data input
function y = fcn(data)

    coder.extrinsic('evalin');

    flag_dead = 0;
    flag_dead = evalin('base', 'flg_dead_v_CP1');

    if flag_dead == 1
        y = 0;
        assignin('base', 'flg_dead_v_CP1', 0);
    else
        y = data;
    end

end

== matlab function CPS_PowerSync_System/Subsystem1/MATLAB Function2 ==
  settings: updateMethod=DISCRETE  sampleTime=0.1
  data: y output
function y = fcn()

    y = 0;
    coder.extrinsic('evalin');

    flag_elected = 0;
    flag_elected = evalin('base', 'flg_elected_CP2'); % Legge la variabile v1 dal Base Workspace

    if flag_elected == 0
        % Significa che il CP 2 non partecipa e deve solo fare da
        % intermediario
        y = 0;
    else if flag_elected == 1
            % Il leader esiste (potrebbe essere il 2 o il 3)
            y = 1;
        end
    end
   
end

== matlab function CPS_PowerSync_System/Subsystem2/MATLAB Function2 ==
  settings: updateMethod=DISCRETE  sampleTime=0.1
  data: y output
function y = fcn()

    y = 0;
    coder.extrinsic('evalin');

    flag_elected = 0;
    flag_elected = evalin('base', 'flg_elected_CP3'); % Legge la variabile v1 dal Base Workspace

    if flag_elected == 0
        % Significa che il CP3 non partecipa e deve solo fare da
        % intermediario
        y = 0;
    else if flag_elected == 1
            % Il leader esiste (potrebbe essere il 2 o il 3)
            y = 1;
        end
    end
   
end

== matlab function CPS_PowerSync_System/Subsystem/MATLAB Function3 ==
  settings: updateMethod=DISCRETE  sampleTime=0.1
  data: data input; w output
function w = readVariable(data)

    coder.extrinsic('evalin');

    w = 0;

    flag_elected = 0;
    flag_elected = evalin('base', 'flg_elected_CP1'); % Legge la variabile v1 dal Base Workspace

    flag_first_instant_w = 0;
    flag_first_instant_w = evalin('base', 'flg_first_instant_w_CP1'); % Legge la variabile v1 dal Base Workspace


    % CI DEVI ANDARE SOLO LA PRIMA VOLTA 
    if flag_elected == 1 && flag_first_instant_w == 1
        w = evalin('base', 'w_CP1');
        assignin('base', 'flg_first_instant_w_CP1', 0);
    else
        assignin('base', 'w_CP1', data);
        w = data;
    end

end

== matlab function CPS_PowerSync_System/Subsystem/MATLAB Function4 ==
  settings: updateMethod=DISCRETE  sampleTime=0.1
  data: y output; data input
function y = fcn(data)

    coder.extrinsic('evalin');

    flag_dead_w = 0;
    flag_dead_w = evalin('base', 'flg_dead_w_CP1');

    if flag_dead_w == 1
        y = 1;
        assignin('base', 'flg_dead_w_CP1', 0);
    else
        y = data;
    end

end

== matlab function CPS_PowerSync_System/Subsystem1/MATLAB Function3 ==
  settings: updateMethod=DISCRETE  sampleTime=0.1
  data: data input; w output
function w = readVariable(data)

    coder.extrinsic('evalin');

    w = 0;

    flag_elected = 0;
    flag_elected = evalin('base', 'flg_elected_CP2'); % Legge la variabile v1 dal Base Workspace

    flag_first_instant_w = 0;
    flag_first_instant_w = evalin('base', 'flg_first_instant_w_CP2'); % Legge la variabile v1 dal Base Workspace


    % CI DEVI ANDARE SOLO LA PRIMA VOLTA 
    if flag_elected == 1 && flag_first_instant_w == 1
        w = evalin('base', 'w_CP2');
        assignin('base', 'flg_first_instant_w_CP2', 0);
    else
        assignin('base', 'w_CP2', data);
        w = data;
    end

end

== matlab function CPS_PowerSync_System/Subsystem1/MATLAB Function4 ==
  settings: updateMethod=DISCRETE  sampleTime=0.1
  data: y output; data input
function y = fcn(data)

    coder.extrinsic('evalin');

    flag_dead_w = 0;
    flag_dead_w = evalin('base', 'flg_dead_w_CP2');

    if flag_dead_w == 1
        y = 1;
        assignin('base', 'flg_dead_w_CP2', 0);
    else
        y = data;
    end

end

== matlab function CPS_PowerSync_System/Subsystem2/MATLAB Function3 ==
  settings: updateMethod=DISCRETE  sampleTime=0.1
  data: data input; w output
function w = readVariable(data)

    coder.extrinsic('evalin');

    w = 0;

    flag_elected = 0;
    flag_elected = evalin('base', 'flg_elected_CP3'); % Legge la variabile v1 dal Base Workspace

    flag_first_instant_w = 0;
    flag_first_instant_w = evalin('base', 'flg_first_instant_w_CP3'); % Legge la variabile v1 dal Base Workspace


    % CI DEVI ANDARE SOLO LA PRIMA VOLTA 
    if flag_elected == 1 && flag_first_instant_w == 1
        w = evalin('base', 'w_CP3');
        assignin('base', 'flg_first_instant_w_CP3', 0);
    else
        assignin('base', 'w_CP3', data);
        w = data;
    end

end

== matlab function CPS_PowerSync_System/Subsystem2/MATLAB Function4 ==
  settings: updateMethod=DISCRETE  sampleTime=0.1
  data: y output; data input
function y = fcn(data)

    coder.extrinsic('evalin');

    flag_dead_w = 0;
    flag_dead_w = evalin('base', 'flg_dead_w_CP3');

    if flag_dead_w == 1
        y = 1;
        assignin('base', 'flg_dead_w_CP3', 0);
    else
        y = data;
    end

end

== matlab function CPS_PowerSync_System/Subsystem/MATLAB Function5 ==
  settings: updateMethod=DISCRETE  sampleTime=0.1
  data: u input; y output
function y = fcn(u)

    coder.extrinsic('evalin');

    flag_reset_w = 0;
    flag_reset_w = evalin('base', 'flg_reset_w_CP1');

    if flag_reset_w == 1
        y = 0;
        assignin('base', 'flg_reset_w_CP1', 0);
    else
        y = u;
    end

end

== matlab function CPS_PowerSync_System/Subsystem/MATLAB Function6 ==
  settings: updateMethod=DISCRETE  sampleTime=0.1
  data: u input; y output
function y = fcn(u)

    coder.extrinsic('evalin');

    flag_reset_v = 0;
    flag_reset_v = evalin('base', 'flg_reset_v_CP1');

    if flag_reset_v == 1
        y = 0;
        assignin('base', 'flg_reset_v_CP1', 0);
    else
        y = u;
    end

end

== matlab function CPS_PowerSync_System/Subsystem1/MATLAB Function5 ==
  settings: updateMethod=DISCRETE  sampleTime=0.1
  data: u input; y output
function y = fcn(u)

    coder.extrinsic('evalin');

    flag_reset_w = 0;
    flag_reset_w = evalin('base', 'flg_reset_w_CP2');

    if flag_reset_w == 1
        y = 0;
        assignin('base', 'flg_reset_w_CP2', 0);
    else
        y = u;
    end

end

== matlab function CPS_PowerSync_System/Subsystem1/MATLAB Function6 ==
  settings: updateMethod=DISCRETE  sampleTime=0.1
  data: u input; y output
function y = fcn(u)

    coder.extrinsic('evalin');

    flag_reset_v = 0;
    flag_reset_v = evalin('base', 'flg_reset_v_CP2');

    if flag_reset_v == 1
        y = 0;
        assignin('base', 'flg_reset_v_CP2', 0);
    else
        y = u;
    end

end

== matlab function CPS_PowerSync_System/Subsystem2/MATLAB Function5 ==
  settings: updateMethod=DISCRETE  sampleTime=0.1
  data: u input; y output
function y = fcn(u)

    coder.extrinsic('evalin');

    flag_reset_w = 0;
    flag_reset_w = evalin('base', 'flg_reset_w_CP3');

    if flag_reset_w == 1
        y = 0;
        assignin('base', 'flg_reset_w_CP3', 0);
    else
        y = u;
    end

end

== matlab function CPS_PowerSync_System/ElecritcVehicles1/Normal.Plugged.Charging/If Action Subsystem/MATLAB Function ==
  data: y output; SoC_EV1 data_store_memory
function y = fcn

global SoC_EV1

y = SoC_EV1;

== matlab function CPS_PowerSync_System/Subsystem2/MATLAB Function6 ==
  settings: updateMethod=DISCRETE  sampleTime=0.1
  data: u input; y output
function y = fcn(u)

    coder.extrinsic('evalin');

    flag_reset_v = 0;
    flag_reset_v = evalin('base', 'flg_reset_v_CP3');

    if flag_reset_v == 1
        y = 0;
        assignin('base', 'flg_reset_v_CP3', 0);
    else
        y = u;
    end

end

== stateflow chart CPS_PowerSync_System/ChargingPoint1 ==
  settings: updateMethod=CONTINUOUS  sampleTime=1
  state Normal
    state Idle
      state Assignment
    state Connected
      state Powering
        state Assignment
      state NotPowering
        state Assignment
      (default) -> (junction 23)
      (junction 23) -> Powering [order 1] : [powerRequest == 1]
      (junction 23) -> NotPowering [order 2]
      NotPowering -> Powering : [powerRequest == 1]
      Powering -> NotPowering : [powerRequest == 0]
    (default) -> (junction 31)
    (junction 31) -> Idle [order 1] : [plug == 0]
    (junction 31) -> Connected [order 2]
    Connected -> Idle : [plug == 0]
    Idle -> Connected : [plug == 1]
  state Error
    state Assignment
  (default) -> Normal
  Normal -> Error : [runPythonScriptRandGen <= (1 - exp((-(elapsed(sec))/300)))]
  Error -> Normal : after(10,sec)
  data: sf_internal_action_state_placeholder_data local double size=1 =0; sf_internal_action_state_placeholder_data local double size=1 =0; sf_internal_action_state_placeholder_data local double size=1 =0; sf_internal_action_state_placeholder_data local double size=1 =0; randUniform function_output; powerRequest input boolean; plug input boolean; enablePowerFlow output boolean
  function randUniform = runPythonScriptRandGen:
    | function randUniform = runPythonScriptRandGen()
    | 
    |     % La funzione è estrinseca, cioè non verrà compilata in codice C.
    |     % Deve essere eseguita come una chiamata MATLAB normale.
    |     coder.extrinsic('pyrunfile');
    | 
    |     % Inizializzo la variabile
    |     randUniform = 0;
    | 
    |     % Esegue lo script Python rand.py e cattura il risultato.
    |     randUniform = pyrunfile("rand.py", "r");
    | end

== matlab function CPS_PowerSync_System/Power supply ==
  settings: updateMethod=DISCRETE  sampleTime=1
  data: y output
function y = power_supply()
    y = 10000;
end

== matlab function CPS_PowerSync_System/MATLAB Function7 ==
  settings: updateMethod=DISCRETE  sampleTime=0.1
  data: actual input; y output; previous input
function y = fcn(actual, previous)

    threshold = 0.001;

    % abs() calcola il valore assoluto
    alfa = abs(actual - previous);

    if alfa < threshold
        y = actual;
    else
        y = 0;
    end


end

== matlab function CPS_PowerSync_System/ElecritcVehicles2/Normal.Plugged.Charging/If Action Subsystem/MATLAB Function ==
  data: y output; SoC_EV2 data_store_memory
function y = fcn

global SoC_EV2

y = SoC_EV2;

== matlab function CPS_PowerSync_System/ElecritcVehicles2/Normal.Plugged.Charging/If Action Subsystem/MATLAB Function1 ==
  settings: updateMethod=DISCRETE
  data: SoC_EV2 data_store_memory; u_current input
function fcn(u_current)

global SoC_EV2

SoC_EV2 = u_current;

== matlab function CPS_PowerSync_System/MATLAB Function8 ==
  settings: updateMethod=DISCRETE  sampleTime=0.1
  data: actual input; y output; previous input
function y = fcn(actual, previous)

    threshold = 0.001;

    % abs() calcola il valore assoluto
    alfa = abs(actual - previous);

    if alfa < threshold
        y = actual;
    else
        y = 0;
    end


end

== matlab function CPS_PowerSync_System/MATLAB Function9 ==
  settings: updateMethod=CONTINUOUS  sampleTime=1
  data: pr_actual_CP2 input; pr_previous_CP2 input
function fcn(pr_actual_CP2, pr_previous_CP2)

    assignin('base', 'pr_previous_CP2', pr_previous_CP2)
    assignin('base', 'pr_actual_CP2', pr_actual_CP2)

end

== matlab function CPS_PowerSync_System/MATLAB Function10 ==
  settings: updateMethod=CONTINUOUS  sampleTime=1
  data: pr_actual_CP1 input; pr_previous_CP1 input
function fcn(pr_actual_CP1, pr_previous_CP1)

    assignin('base', 'pr_previous_CP1', pr_previous_CP1)
    assignin('base', 'pr_actual_CP1', pr_actual_CP1)

end

== matlab function CPS_PowerSync_System/ElecritcVehicles2/Normal.Plugged.Completed/If Action Subsystem/MATLAB Function ==
  data: y output; SoC_EV2 data_store_memory
function y = fcn

global SoC_EV2

y = SoC_EV2;

== matlab function CPS_PowerSync_System/MATLAB Function11 ==
  settings: updateMethod=CONTINUOUS  sampleTime=1
  data: pr_actual_CP3 input; pr_previous_CP3 input
function fcn(pr_actual_CP3, pr_previous_CP3)

    assignin('base', 'pr_previous_CP3', pr_previous_CP3)
    assignin('base', 'pr_actual_CP3', pr_actual_CP3)

end

== matlab function CPS_PowerSync_System/MATLAB Function4 ==
  settings: updateMethod=DISCRETE  sampleTime=0.1
  data: actual input; y output; previous input
function y = fcn(actual, previous)

    threshold = 0.001;

    % abs() calcola il valore assoluto
    alfa = abs(actual - previous);

    if alfa < threshold
        y = actual;
    else
        y = 0;
    end


end

== matlab function CPS_PowerSync_System/ElecritcVehicles2/Normal.Plugged.Completed/If Action Subsystem/MATLAB Function1 ==
  settings: updateMethod=DISCRETE
  data: SoC_EV2 data_store_memory; u input
function fcn(u)

global SoC_EV2

SoC_EV2 = u;
